simulink model "MBD_Math_Operations_2"  (R2021b)
settings: Solver=FixedStepDiscrete  StartTime=0.0  StopTime=10.0  FixedStep=0.0001  RelTol=1e-3
libraries: simulink x2
settings Model: Creator=waleed.elshemy  LastModifiedBy=waleed.elshemy
settings OptimizationCC: DefaultParameterBehavior=Inlined  UseDivisionForNetSlopeComputation=on  GainParamInheritBuiltInType=on  UseFloatMulNetSlope=on  InlineInvariantSignals=on  PassReuseOutputArgsAs=Individual arguments  ZeroExternalMemoryAtStartup=off  ZeroInternalMemoryAtStartup=off  NoFixptDivByZeroProtection=on  EfficientFloat2IntCast=on  LifeSpan=1  OptimizeBlockOrder=speed  DifferentSizesBufferReuse=on  EfficientTunableParamExpr=on
settings DebuggingCC: ParameterTunabilityLossMsg=error
settings HardwareCC: ProdLongLongMode=on
settings SFSimCC: MATLABDynamicMemAlloc=off
settings RTWCC: Description=Embedded Coder  SystemTargetFile=ert.tlc  TemplateMakefile=ert_default_tmf
settings CodeAppCC: ForceParamTrailComments=on  IgnoreCustomStorageClasses=off  OperatorAnnotations=on  SimulinkDataObjDesc=on  SFDataObjDesc=on  CustomSymbolStrGlobalVar=rt$N$M  CustomSymbolStrType=$N$M  CustomSymbolStrFcn=$N$M$F  CustomSymbolStrMacro=$N$M  InsertBlockDesc=on
settings ERTTargetCC: TargetLangStandard=C99 (ISO)  GenerateSampleERTMain=on  IncludeMdlTerminateFcn=off  CombineSignalStateStructs=on  SupportComplex=off  SupportContinuousTime=on  InlinedParameterPlacement=NonHierarchical  ERTCustomFileTemplate=example_file_process.tlc  ERTFilePackagingFormat=CompactWithDataFile

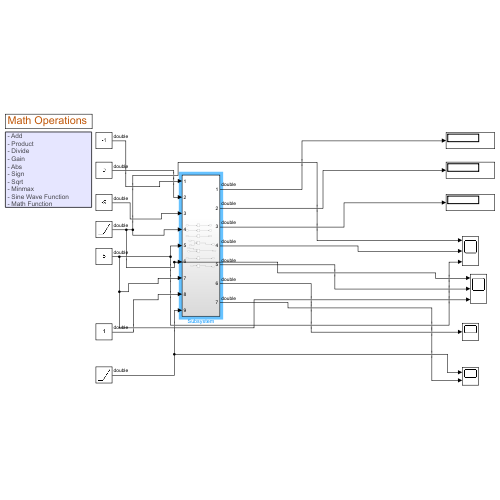
[thumbnail: Simulink's stored preview of the top-level diagram]
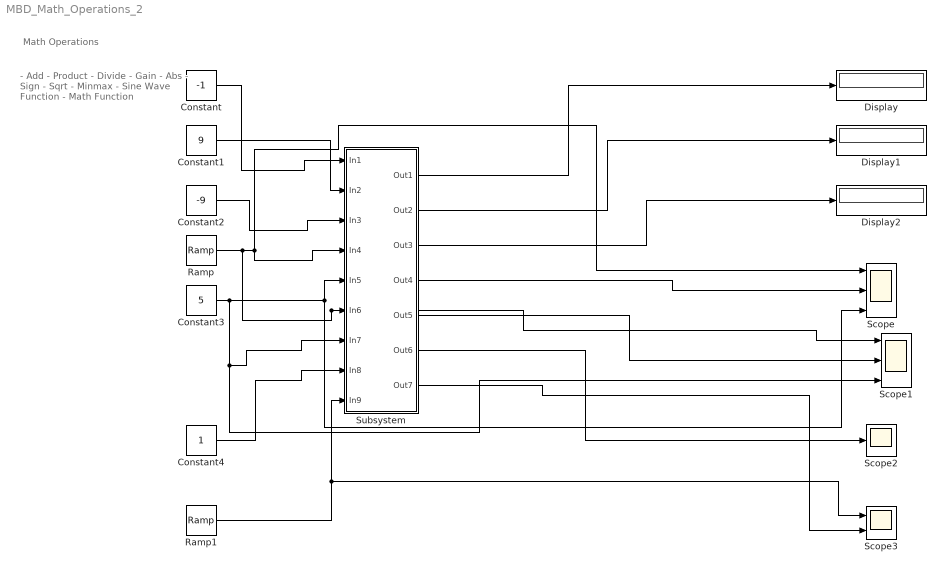
== system MBD_Math_Operations_2 ==
  note: - Add
      | - Product
      | - Divide
      | - Gain
      | - Abs
      | - Sign
      | - Sqrt
      | - Minmax
      | - Sine Wave Function
      | - Math Function
  note: Math Operations
  Constant : Constant  Value=-1
  Constant1 : Constant  Value=9
  Constant2 : Constant  Value=-9
  Constant3 : Constant  Value=5
  Constant4 : Constant
  Display : Display
  Display1 : Display
  Display2 : Display
  Ramp : simulink/Sources/Ramp  slope=1  start=0  InitialOutput=0
  Ramp1 : simulink/Sources/Ramp  slope=1  start=0  InitialOutput=0
  Scope : Scope  NumInputPorts=3
  Scope1 : Scope  NumInputPorts=3
  Scope2 : Scope
  Scope3 : Scope  NumInputPorts=2
  Subsystem : Subsystem
  wires:
  Ramp/1 -> Scope1/1, Subsystem/6(In6), Subsystem/4(In4), Scope/1
  Constant3/1 -> Subsystem/7(In7), Scope1/3, Subsystem/5(In5), Scope/3
  Ramp1/1 -> Subsystem/9(In9), Scope3/1
  Constant/1 -> Subsystem/1(In1)
  Constant1/1 -> Subsystem/2(In2)
  Constant2/1 -> Subsystem/3(In3)
  Constant4/1 -> Subsystem/8(In8)
  Subsystem/1(Out1) -> Display/1
  Subsystem/2(Out2) -> Display1/1
  Subsystem/3(Out3) -> Display2/1
  Subsystem/4(Out4) -> Scope/2
  Subsystem/5(Out5) -> Scope1/2
  Subsystem/6(Out6) -> Scope2/1
  Subsystem/7(Out7) -> Scope3/2

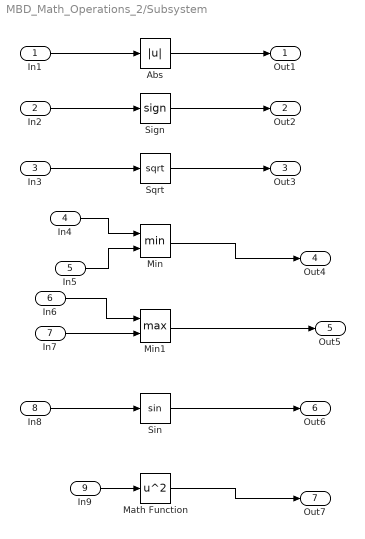
== system MBD_Math_Operations_2/Subsystem ==
  In1 : Inport
  In2 : Inport  Port=2
  In3 : Inport  Port=3
  In4 : Inport  Port=4
  In5 : Inport  Port=5
  In6 : Inport  Port=6
  In7 : Inport  Port=7
  In8 : Inport  Port=8
  In9 : Inport  Port=9
  Abs : Abs
  Math Function : Math  Operator=square  SaturateOnIntegerOverflow=on
  Min : MinMax  Inputs=2
  Min1 : MinMax  Function=max  Inputs=2
  Sign : Signum
  Sin : Trigonometry
  Sqrt : Sqrt  SaturateOnIntegerOverflow=on
  Out1 : Outport
  Out2 : Outport  Port=2
  Out3 : Outport  Port=3
  Out4 : Outport  Port=4
  Out5 : Outport  Port=5
  Out6 : Outport  Port=6
  Out7 : Outport  Port=7
  wires:
  In7/1 -> Min1/2
  In2/1 -> Sign/1
  Sign/1 -> Out2/1
  In1/1 -> Abs/1
  In6/1 -> Min1/1
  Sqrt/1 -> Out3/1
  Min1/1 -> Out5/1
  Math Function/1 -> Out7/1
  In8/1 -> Sin/1
  In9/1 -> Math Function/1
  In4/1 -> Min/1
  In5/1 -> Min/2
  Min/1 -> Out4/1
  In3/1 -> Sqrt/1
  Sin/1 -> Out6/1
  Abs/1 -> Out1/1
